simulink model "Lab9_simulink"  (Simulink 7.3)
settings: Solver=ode45  StartTime=0.0  StopTime=10.0  RelTol=1e-3
undefined symbols (not defined in the file or in its folder): get, i
libraries: commsink2 x7, commdigbbndpm3 x3, commdigbbndcpm2 x2, commrandsrc2 x1, commdigbbndam3 x1, commdigbbndfm2 x1
settings Model: Creator=user_ftk10  LastModifiedBy=user_ftk10

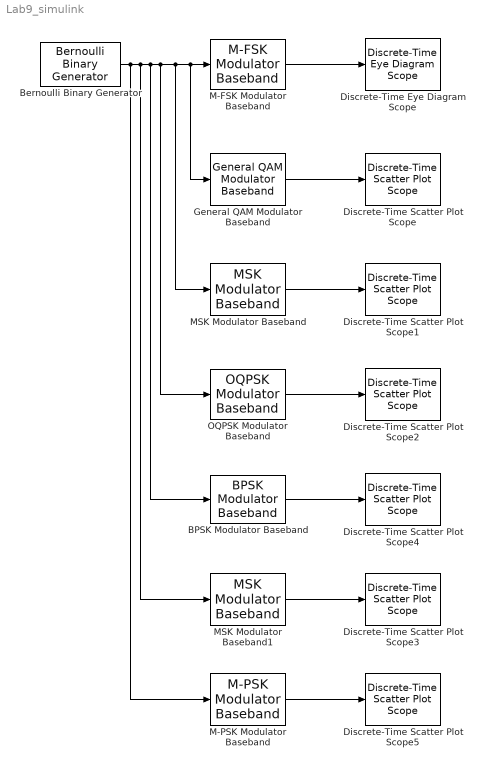
== system Lab9_simulink ==
  BPSK Modulator Baseband : commdigbbndpm3/BPSK Modulator Baseband  DialogController=commDDGCreate  DialogControllerArgs=DataTag0  SystemSampleTime=-1  Ph=0  outDtype=double  outWordLen=16  outUDDataType=sfix(16)  outFracLenMode=Best precision  outFracLen=15
  Bernoulli Binary Generator : commrandsrc2/Bernoulli Binary Generator  DialogController=commDDGCreate  DialogControllerArgs=DataTag1  SystemSampleTime=-1  P=0.5  seed=61  Ts=1  frameBased=off  sampPerFrame=1  orient=off  outDataType=double
  Discrete-Time Eye Diagram Scope : commsink2/Discrete-Time Eye Diagram Scope  Tag=EyeDiagram  SystemSampleTime=-1  sampPerSymb=8  offsetEye=0  symbPerTrace=1  numTraces=40  numNewFrames=10  LineStyles=-  LineColors=b  dupPoints=on  fading=on  render=on  AxisGrid=on  yMin=-3.15  yMax=3.15  inphaseLabel=In-phase Amplitude  quadratureLabel=Quadrature Amplitude  openScopeAtSimStart=on  dispDiagram=In-phase and Quadrature  FrameNumber=off  FigPos=get(0,'defaultfigureposition');  figTitle=Eye Diagram  block_type_=eye  numLinesMax=8
  Discrete-Time Scatter Plot Scope{,1..5} (6 alike) : commsink2/Discrete-Time Scatter Plot Scope  Tag=ScatterPlot  SystemSampleTime=-1  sampPerSymb=1  offsetEye=0  numTraces=40  numNewFrames=10  LineMarkers=.  LineColors=b  fading=on  render=on  AxisGrid=on  xMin=-3.3  xMax=3.315  yMin=-3.3  yMax=3.315  inphaseLabel=In-phase Amplitude  quadratureLabel=Quadrature Amplitude  openScopeAtSimStart=on  FrameNumber=off  FigPos=get(0,'defaultfigureposition');  figTitle=Scatter Plot  numLinesMax=8  block_type_=scatter
  General QAM Modulator Baseband : commdigbbndam3/General QAM Modulator Baseband  DialogController=commDDGCreate  DialogControllerArgs=DataTag2  SigCon=[exp(2*pi*i*[0:7]/8)]  outDtype=double  outWordLen=16  outUDDataType=sfix(16)  outFracLenMode=Best precision  outFracLen=15
  M-FSK Modulator Baseband : commdigbbndfm2/M-FSK Modulator Baseband  M=8  InType=Integer  Enc=Binary  freqSep=6  phaseType=Continuous  numSamp=17  outDataType=double
  M-PSK Modulator Baseband : commdigbbndpm3/M-PSK Modulator Baseband  DialogController=commDDGCreate  DialogControllerArgs=DataTag3  M=8  InType=Integer  Enc=Binary  Mapping=[0:7]  Ph=pi/8  outDtype=double  outWordLen=16  outUDDataType=sfix(16)  outFracLenMode=Best precision  outFracLen=15
  MSK Modulator Baseband : commdigbbndcpm2/MSK Modulator Baseband  SystemSampleTime=-1  inputType=Integer  phaseOffset=0  samplesPerSymbol=8  outDataType=double
  MSK Modulator Baseband1 : commdigbbndcpm2/MSK Modulator Baseband  SystemSampleTime=-1  inputType=Integer  phaseOffset=0  samplesPerSymbol=8  outDataType=double
  OQPSK Modulator Baseband : commdigbbndpm3/OQPSK Modulator Baseband  DialogController=commDDGCreate  DialogControllerArgs=DataTag4  InType=Integer  Ph=0  outDtype=double  outWordLen=16  outUDDataType=sfix(16)  outFracLenMode=Best precision  outFracLen=15
  wires:
  Bernoulli Binary Generator/1 -> M-FSK Modulator Baseband/1, General QAM Modulator Baseband/1, MSK Modulator Baseband/1, OQPSK Modulator Baseband/1, BPSK Modulator Baseband/1, MSK Modulator Baseband1/1, M-PSK Modulator Baseband/1
  M-FSK Modulator Baseband/1 -> Discrete-Time Eye Diagram Scope/1
  General QAM Modulator Baseband/1 -> Discrete-Time Scatter Plot Scope/1
  MSK Modulator Baseband/1 -> Discrete-Time Scatter Plot Scope1/1
  M-PSK Modulator Baseband/1 -> Discrete-Time Scatter Plot Scope5/1
  MSK Modulator Baseband1/1 -> Discrete-Time Scatter Plot Scope3/1
  BPSK Modulator Baseband/1 -> Discrete-Time Scatter Plot Scope4/1
  OQPSK Modulator Baseband/1 -> Discrete-Time Scatter Plot Scope2/1
